simulink model "Lab_07_Task_03"  (R2023b)
settings: Solver=VariableStepAuto  StartTime=0.0  StopTime=10.0  RelTol=1e-3
StopFcn:
  | subplot(2,1,1)
  | plot(out.simout1)
  | 
  | subplot(2,1,2)
  | plot(out.simout)
libraries: dspsnks4 x1, dspvision x1
settings Model: Creator=Osii  LastModifiedBy=Azlaan
settings OptimizationCC: ReuseModelBlockBuffer=off

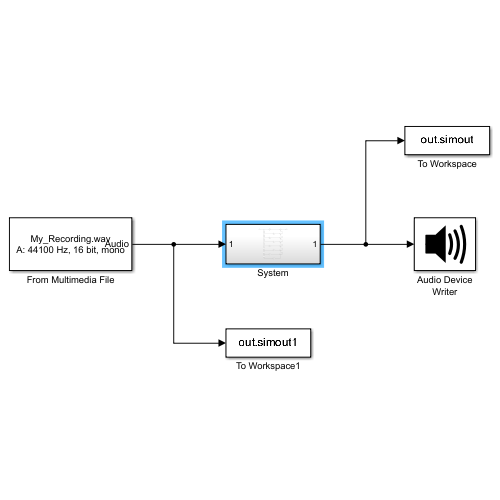
[thumbnail: Simulink's stored preview of the top-level diagram]
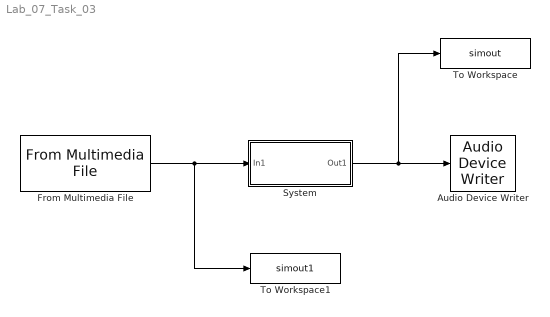
== system Lab_07_Task_03 ==
  Audio Device Writer : dspsnks4/Audio Device Writer  Driver=DirectSound  Device=Default  InheritSampleRate=on  SampleRate=8000  BitDepth=16-bit integer  BufferSize=4096  NumBuffers=10  DefaultOutputChannelMapping=on  OutputChannelMapping=1:2  OutputNumUnderrunSamples=off  DriverIdx=1  DeviceWarnFlag=''
  From Multimedia File : dspvision/From Multimedia File  inputFilename=D:\NUST EME\5th Semester\Signals_Systems\Lab\Lab 7\My_Recording.wav  readRange=[1 Inf]  loop=on  numPlays=inf  outputStreams=Audio only  videoDataType=single  audioDataType=double  inheritSampleTime=on  userDefinedSampleTime=1/30  noAudioOutput=off  isIntensityVideo=off  fourcc=RGB  colorVideoFormat=Separate color signals  outputEOF=off  dataOrg=Column-major  audioFrameSize=1024  computeAudioFrameSize=off  outSamplingMode=Sample based
      settings: LibrarySourceBlock=audiosources/From Multimedia File
  System : Subsystem
  To Workspace : ToWorkspace  VariableName=simout  SaveFormat=Timeseries  SampleTime=-1
  To Workspace1 : ToWorkspace  VariableName=simout1  SaveFormat=Timeseries  SampleTime=-1
  wires:
  From Multimedia File/1 -> To Workspace1/1, System/1(In1)
  System/1(Out1) -> To Workspace/1, Audio Device Writer/1

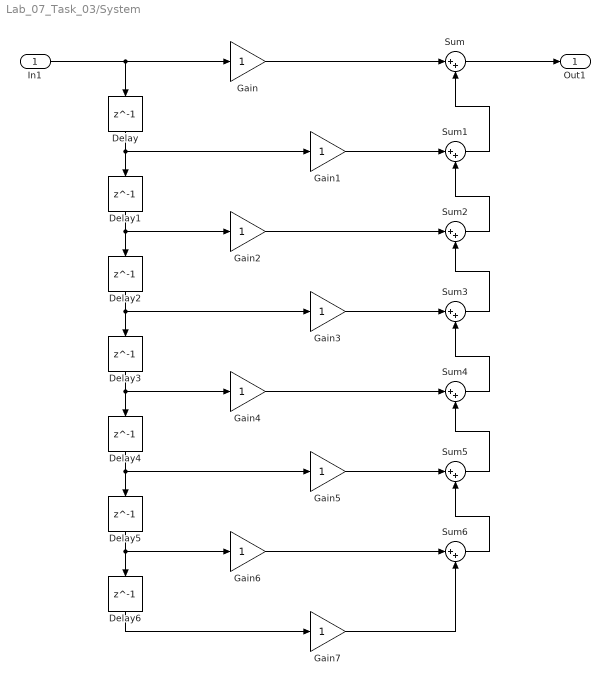
== system Lab_07_Task_03/System ==
  In1 : Inport
  Delay{,1..6} (7 alike) : Delay  DelayLength=1  InputProcessing=Columns as channels (frame based)
  Gain{,1..7} (8 alike) : Gain
  Sum{,1..6} (7 alike) : Sum  Inputs=|++
  Out1 : Outport
  wires:
  In1/1 -> Delay/1, Gain/1
  Delay2/1 -> Gain3/1, Delay3/1
  Delay/1 -> Delay1/1, Gain1/1
  Delay3/1 -> Gain4/1, Delay4/1
  Delay4/1 -> Gain5/1, Delay5/1
  Delay5/1 -> Gain6/1, Delay6/1
  Gain/1 -> Sum/1
  Sum/1 -> Out1/1
  Delay1/1 -> Gain2/1, Delay2/1
  Gain1/1 -> Sum1/1
  Gain3/1 -> Sum3/1
  Gain5/1 -> Sum5/1
  Gain4/1 -> Sum4/1
  Gain6/1 -> Sum6/1
  Delay6/1 -> Gain7/1
  Sum6/1 -> Sum5/2
  Sum5/1 -> Sum4/2
  Sum4/1 -> Sum3/2
  Sum3/1 -> Sum2/2
  Gain2/1 -> Sum2/1
  Sum2/1 -> Sum1/2
  Sum1/1 -> Sum/2
  Gain7/1 -> Sum6/2
